simulink model "sampleModel1637"  (R2023a)
settings: Solver=VariableStepAuto  StartTime=0.0  StopTime=10.0  RelTol=1e-3
libraries: hdlsllib x7, simulink x3
settings Model: Creator=user1  LastModifiedBy=user1

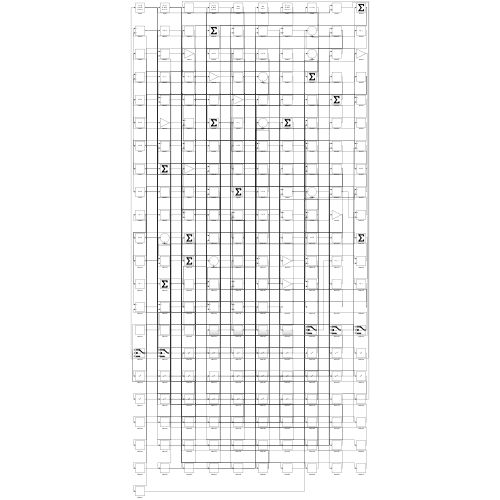
[thumbnail: Simulink's stored preview of the top-level diagram]
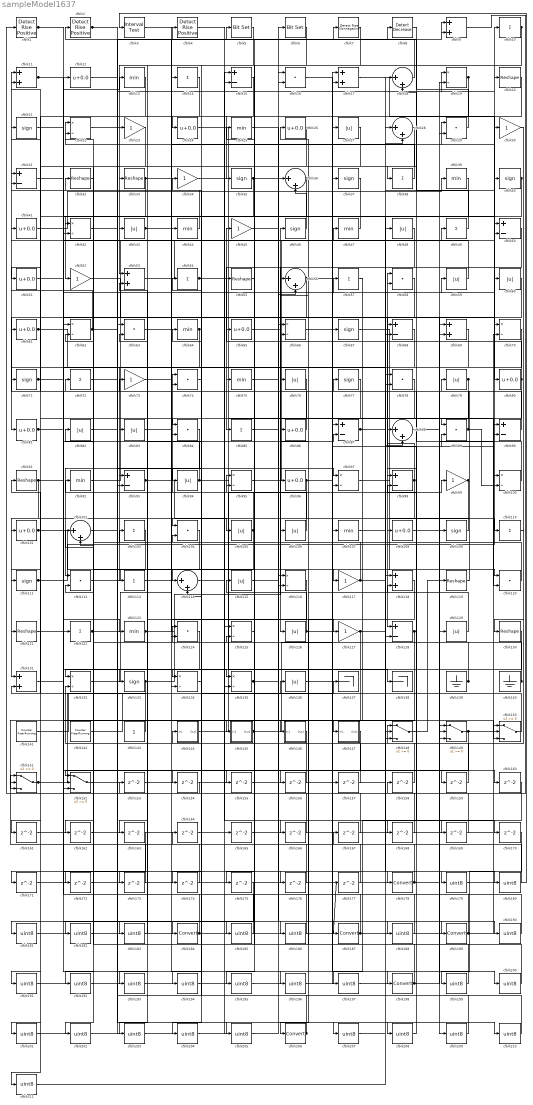
== system sampleModel1637 ==
  cfblk1 : hdlsllib/Logic and Bit Operations/Detect Rise Positive  vinit=0  OutDataTypeStr=boolean
  cfblk{10,14,38,49,54,57,72,85,103,110,113,122} (12 alike) : Sum  Inputs=+
  cfblk{19,22,42,62,66,70,95,97,100,116,125,132,134..135} (14 alike) : Product  Inputs=*/  RndMeth=Zero  SaturateOnIntegerOverflow=on
  cfblk{12,24,26,41,51,61,65,80..81,86,96,101,108} (13 alike) : Bias  Bias=0.0  SaturateOnIntegerOverflow=off
  cfblk{18,28,36,56,88,102,114} (7 alike) : Sum  Inputs=|++
  cfblk{16,29,58,63,74,78,84,89,104,112,120,124} (12 alike) : DotProduct  OutDataTypeStr=Inherit: Inherit via internal rule
  cfblk{27,43,48,59..60,76,79,82..83,94,105..106,115,126,129,136} (16 alike) : Abs  SaturateOnIntegerOverflow=off
  cfblk{13,25,39,44,47,64,75,92,107,123} (10 alike) : MinMax
  cfblk{21,35,37,40,46,67,71,77,109,111,133} (11 alike) : Signum
  cfblk{9,11,17,53,69,118,131} (7 alike) : Sum
  cfblk{23,30,34,45,52,73,99,117,127} (9 alike) : Gain
  cfblk{20,32..33,55,91,119,121,130} (8 alike) : Reshape
  cfblk{15,31,50,68,87,90,93,98,128} (9 alike) : Sum  Inputs=+-
  cfblk137 : Terminator
  cfblk138 : Terminator
  cfblk139 : Ground
  cfblk140 : Ground
  cfblk141 : hdlsllib/Sources/Counter Free-Running  NumBits=16  tsamp=-1
  cfblk142 : hdlsllib/Sources/Counter Free-Running  NumBits=16  tsamp=-1
  cfblk143 : Constant  SampleTime=-1
  cfblk144 : Subsystem
      settings: LibrarySourceBlock=|
      | hdlsllib/Ports &
      | Subsystems/Subsystem
  cfblk145 : Subsystem
      settings: LibrarySourceBlock=|
      | hdlsllib/Ports &
      | Subsystems/Subsystem
  cfblk146 : Subsystem
      settings: LibrarySourceBlock=|
      | hdlsllib/Ports &
      | Subsystems/Subsystem
  cfblk147 : Subsystem
      settings: LibrarySourceBlock=|
      | hdlsllib/Ports &
      | Subsystems/Subsystem
  cfblk{148..152} (5 alike) : Switch  SaturateOnIntegerOverflow=off  InputSameDT=off
  cfblk{153..177} (25 alike) : Delay  SampleTime=1
  cfblk{178,184,187,189,198,206} (6 alike) : DataTypeConversion  SaturateOnIntegerOverflow=off  RndMeth=Floor
  cfblk{179..183,185..186,188,190..197,199..205,207..211} (28 alike) : DataTypeConversion  OutDataTypeStr=uint8  SaturateOnIntegerOverflow=off  RndMeth=Floor
  cfblk2 : hdlsllib/Logic and Bit Operations/Detect Rise Positive  vinit=0  OutDataTypeStr=boolean
  cfblk3 : hdlsllib/Logic and Bit Operations/Interval Test  IntervalClosedRight=on  uplimit=0.5  IntervalClosedLeft=on  lowlimit=-0.5  OutDataTypeStr=boolean
  cfblk4 : hdlsllib/Logic and Bit Operations/Detect Rise Positive  vinit=0  OutDataTypeStr=boolean
  cfblk5 : simulink/Logic and Bit Operations/Bit Set  iBit=0
      settings: LibrarySourceBlock=|
      | hdlsllib/Logic and Bit
      | Operations/Bit Set
  cfblk6 : simulink/Logic and Bit Operations/Bit Set  iBit=0
      settings: LibrarySourceBlock=|
      | hdlsllib/Logic and Bit
      | Operations/Bit Set
  cfblk7 : hdlsllib/Logic and Bit Operations/Detect Rise Nonnegative  vinit=0  OutDataTypeStr=boolean
  cfblk8 : simulink/Logic and Bit Operations/Detect Decrease  vinit=0.0  OutDataTypeStr=boolean
      settings: LibrarySourceBlock=|
      | hdlsllib/Logic and Bit
      | Operations/Detect
      | Decrease
  wires:
  cfblk92/1 -> cfblk47/1
  cfblk14/1 -> cfblk53/1
  cfblk148/1 -> cfblk119/1
  cfblk112/1 -> cfblk114/1
  cfblk81/1 -> cfblk60/1, cfblk190/1
  cfblk111/1 -> cfblk10/1, cfblk50/2
  cfblk97/1 -> cfblk120/1
  cfblk74/1 -> cfblk131/1
  cfblk134/1 -> cfblk34/1
  cfblk95/1 -> cfblk58/1
  cfblk64/1 -> cfblk113/1, cfblk171/1
  cfblk141/1 -> cfblk17/1
  cfblk48/1 -> cfblk126/1
  cfblk30/1 -> cfblk148/1
  cfblk101/1 -> cfblk149/1, cfblk176/1
  cfblk41/1 -> cfblk39/1
  cfblk144/1(Out1) -> cfblk99/1
  cfblk6/1 -> cfblk33/1
  cfblk66/1 -> cfblk198/1
  cfblk149/1 -> cfblk100/1, cfblk156/1
  cfblk54/1 -> cfblk138/1, cfblk170/1
  cfblk53/1 -> cfblk49/1
  cfblk94/1 -> cfblk117/1, cfblk73/1
  cfblk56/1 -> cfblk81/1, cfblk149/3
  cfblk143/1 -> cfblk91/1
  cfblk91/1 -> cfblk121/1, cfblk13/1
  cfblk76/1 -> cfblk111/1
  cfblk50/1 -> cfblk85/1
  cfblk98/1 -> cfblk58/2, cfblk108/1
  cfblk15/1 -> cfblk43/1
  cfblk133/1 -> cfblk46/1, cfblk131/2
  cfblk152/1 -> cfblk37/1
  cfblk10/1 -> cfblk83/1, cfblk75/1
  cfblk79/1 -> cfblk149/2, cfblk154/1
  cfblk123/1 -> cfblk96/1, cfblk30/1
  cfblk127/1 -> cfblk150/2, cfblk181/1
  cfblk29/1 -> cfblk2/1
  cfblk150/1 -> cfblk54/1
  cfblk146/1(Out1) -> cfblk144/1(In1)
  cfblk63/1 -> cfblk44/1
  cfblk2/1 -> cfblk145/1(In1), cfblk97/2, cfblk186/1
  cfblk36/1 -> cfblk52/1, cfblk185/1
  cfblk62/1 -> cfblk11/1, cfblk4/1
  cfblk8/1 -> cfblk38/1
  cfblk126/1 -> cfblk115/1, cfblk89/2, cfblk90/2
  cfblk117/1 -> cfblk86/1, cfblk169/1
  cfblk132/1 -> cfblk14/1
  cfblk67/1 -> cfblk110/1
  cfblk16/1 -> cfblk189/1
  cfblk82/1 -> cfblk20/1
  cfblk85/1 -> cfblk57/1
  cfblk17/1 -> cfblk80/1
  cfblk38/1 -> cfblk22/1
  cfblk93/1 -> cfblk105/1, cfblk200/1
  cfblk60/1 -> cfblk128/1
  cfblk99/1 -> cfblk174/1, cfblk175/1
  cfblk84/1 -> cfblk112/1
  cfblk86/1 -> cfblk31/1
  cfblk109/1 -> cfblk104/1
  cfblk34/1 -> cfblk120/2
  cfblk5/1 -> cfblk24/1
  cfblk39/1 -> cfblk98/1
  cfblk27/1 -> cfblk61/1
  cfblk120/1 -> cfblk64/1
  cfblk80/1 -> cfblk45/1, cfblk161/1
  cfblk140/1 -> cfblk74/1, cfblk92/1
  cfblk51/1 -> cfblk62/1
  cfblk131/1 -> cfblk12/1
  cfblk145/1(Out1) -> cfblk67/1, cfblk56/2
  cfblk90/1 -> cfblk11/2
  cfblk1/1 -> cfblk122/1, cfblk50/1, cfblk68/1
  cfblk24/1 -> cfblk128/2
  cfblk104/1 -> cfblk133/1
  cfblk114/1 -> cfblk15/1
  cfblk119/1 -> cfblk79/1
  cfblk61/1 -> cfblk76/1, cfblk173/1
  cfblk122/1 -> cfblk8/1, cfblk150/3
  cfblk128/1 -> cfblk151/3, cfblk98/2
  cfblk115/1 -> cfblk59/1
  cfblk106/1 -> cfblk62/2
  cfblk55/1 -> cfblk5/1
  cfblk96/1 -> cfblk17/2, cfblk162/1
  cfblk13/1 -> cfblk51/1
  cfblk52/1 -> cfblk129/1
  cfblk73/1 -> cfblk9/1
  cfblk65/1 -> cfblk27/1
  cfblk89/1 -> cfblk31/2, cfblk100/2
  cfblk113/1 -> cfblk127/1
  cfblk59/1 -> cfblk41/1
  cfblk43/1 -> cfblk135/1, cfblk9/2, cfblk70/1
  cfblk31/1 -> cfblk123/1
  cfblk20/1 -> cfblk35/1
  cfblk139/1 -> cfblk124/1, cfblk134/1
  cfblk3/1 -> cfblk178/1
  cfblk33/1 -> cfblk29/1, cfblk152/3, cfblk68/2
  cfblk44/1 -> cfblk21/1
  cfblk47/1 -> cfblk42/1
  cfblk151/1 -> cfblk137/1, cfblk87/2
  cfblk57/1 -> cfblk147/1(In1)
  cfblk100/1 -> cfblk77/1
  cfblk46/1 -> cfblk36/2
  cfblk121/1 -> cfblk135/2
  cfblk35/1 -> cfblk89/1, cfblk94/1
  cfblk142/1 -> cfblk55/1
  cfblk25/1 -> cfblk187/1
  cfblk40/1 -> cfblk93/1, cfblk71/1, cfblk101/1
  cfblk110/1 -> cfblk130/1
  cfblk102/1 -> cfblk184/1
  cfblk118/1 -> cfblk206/1
  cfblk75/1 -> cfblk19/1
  cfblk18/1 -> cfblk7/1
  cfblk135/1 -> cfblk95/2, cfblk188/1
  cfblk108/1 -> cfblk90/1
  cfblk105/1 -> cfblk74/2, cfblk124/2
  cfblk71/1 -> cfblk42/2, cfblk146/1(In1)
  cfblk26/1 -> cfblk132/1
  cfblk129/1 -> cfblk26/1
  cfblk7/1 -> cfblk84/1
  cfblk68/1 -> cfblk93/2
  cfblk87/1 -> cfblk78/1, cfblk40/1
  cfblk42/1 -> cfblk97/1
  cfblk136/1 -> cfblk148/3
  cfblk11/1 -> cfblk78/2, cfblk159/1
  cfblk19/1 -> cfblk134/2, cfblk168/1
  cfblk49/1 -> cfblk18/2
  cfblk32/1 -> cfblk152/1
  cfblk125/1 -> cfblk95/1
  cfblk153/1 -> cfblk15/2
  cfblk154/1 -> cfblk1/1
  cfblk77/1 -> cfblk155/1
  cfblk155/1 -> cfblk148/2
  cfblk156/1 -> cfblk63/2
  cfblk157/1 -> cfblk104/2
  cfblk9/1 -> cfblk158/1
  cfblk158/1 -> cfblk53/2
  cfblk159/1 -> cfblk132/2
  cfblk45/1 -> cfblk160/1
  cfblk161/1 -> cfblk70/2
  cfblk37/1 -> cfblk163/1
  cfblk164/1 -> cfblk18/1
  cfblk165/1 -> cfblk29/2
  cfblk4/1 -> cfblk166/1
  cfblk166/1 -> cfblk22/2
  cfblk167/1 -> cfblk87/1
  cfblk168/1 -> cfblk56/1
  cfblk169/1 -> cfblk114/2
  cfblk171/1 -> cfblk19/2
  cfblk147/1(Out1) -> cfblk172/1
  cfblk172/1 -> cfblk36/1
  cfblk173/1 -> cfblk112/2
  cfblk174/1 -> cfblk151/2
  cfblk176/1 -> cfblk151/1
  cfblk177/1 -> cfblk84/2
  cfblk178/1 -> cfblk167/1, cfblk106/1
  cfblk83/1 -> cfblk179/1
  cfblk179/1 -> cfblk3/1
  cfblk107/1 -> cfblk180/1
  cfblk180/1 -> cfblk82/1
  cfblk181/1 -> cfblk107/1
  cfblk103/1 -> cfblk182/1
  cfblk182/1 -> cfblk48/1
  cfblk130/1 -> cfblk183/1
  cfblk183/1 -> cfblk103/1
  cfblk184/1 -> cfblk177/1, cfblk152/2, cfblk150/1
  cfblk185/1 -> cfblk102/1
  cfblk186/1 -> cfblk102/2
  cfblk187/1 -> cfblk153/1, cfblk136/1
  cfblk188/1 -> cfblk25/1
  cfblk189/1 -> cfblk125/2, cfblk32/1
  cfblk190/1 -> cfblk16/1
  cfblk163/1 -> cfblk191/1
  cfblk191/1 -> cfblk16/2
  cfblk69/1 -> cfblk192/1
  cfblk192/1 -> cfblk157/1
  cfblk78/1 -> cfblk193/1
  cfblk193/1 -> cfblk69/1
  cfblk58/1 -> cfblk194/1
  cfblk194/1 -> cfblk69/2
  cfblk28/1 -> cfblk195/1
  cfblk195/1 -> cfblk109/1
  cfblk21/1 -> cfblk196/1
  cfblk196/1 -> cfblk28/1
  cfblk160/1 -> cfblk197/1
  cfblk197/1 -> cfblk28/2
  cfblk198/1 -> cfblk65/1, cfblk72/1
  cfblk170/1 -> cfblk199/1
  cfblk199/1 -> cfblk66/1
  cfblk200/1 -> cfblk66/2
  cfblk23/1 -> cfblk201/1
  cfblk201/1 -> cfblk165/1
  cfblk124/1 -> cfblk202/1
  cfblk202/1 -> cfblk23/1
  cfblk116/1 -> cfblk203/1
  cfblk203/1 -> cfblk6/1
  cfblk70/1 -> cfblk204/1
  cfblk204/1 -> cfblk116/1
  cfblk162/1 -> cfblk205/1
  cfblk205/1 -> cfblk116/2
  cfblk206/1 -> cfblk164/1, cfblk125/1
  cfblk12/1 -> cfblk207/1
  cfblk207/1 -> cfblk118/1
  cfblk72/1 -> cfblk208/1
  cfblk208/1 -> cfblk118/2
  cfblk88/1 -> cfblk209/1
  cfblk209/1 -> cfblk63/1
  cfblk22/1 -> cfblk210/1
  cfblk210/1 -> cfblk88/1
  cfblk175/1 -> cfblk211/1
  cfblk211/1 -> cfblk88/2

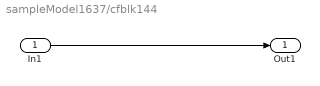
== system sampleModel1637/cfblk144 ==
  In1 : Inport
  Out1 : Outport
  wires:
  In1/1 -> Out1/1

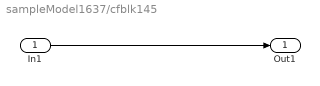
== system sampleModel1637/cfblk145 ==
  In1 : Inport
  Out1 : Outport
  wires:
  In1/1 -> Out1/1

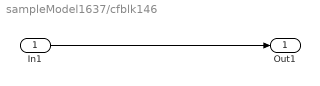
== system sampleModel1637/cfblk146 ==
  In1 : Inport
  Out1 : Outport
  wires:
  In1/1 -> Out1/1

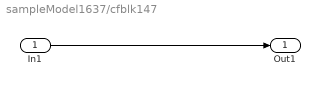
== system sampleModel1637/cfblk147 ==
  In1 : Inport
  Out1 : Outport
  wires:
  In1/1 -> Out1/1
